simulink model "lab0_tutorial_simulink_model"  (R2021b)
settings: Solver=VariableStepAuto  StartTime=0.0  StopTime=10.0  RelTol=1e-3
settings Model: Creator=rcmas  LastModifiedBy=rcmas

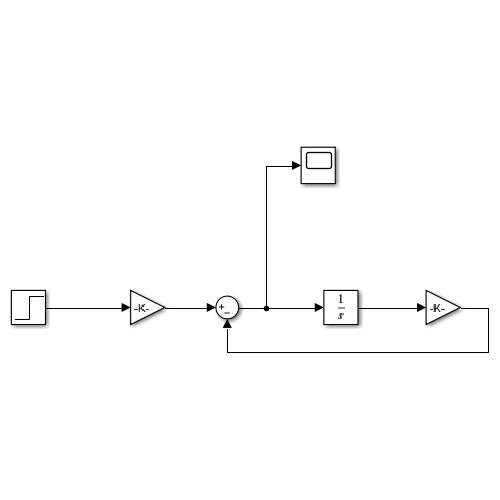
[thumbnail: Simulink's stored preview of the top-level diagram]
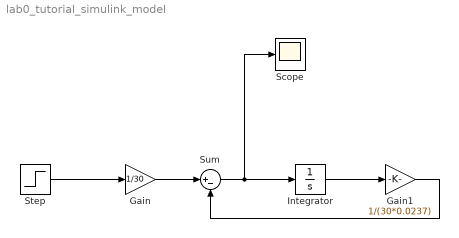
== system lab0_tutorial_simulink_model ==
  Gain : Gain  Gain=1/30
  Gain1 : Gain  Gain=1/(30*0.0237)
  Integrator : Integrator
  Scope : Scope
  Step : Step  SampleTime=0
  Sum : Sum  Inputs=|+-
  wires:
  Step/1 -> Gain/1
  Gain/1 -> Sum/1
  Sum/1 -> Scope/1, Integrator/1
  Integrator/1 -> Gain1/1
  Gain1/1 -> Sum/2
